simulink model "uz_d_inverter_adapter"  (R2024b)
settings: Solver=FixedStepDiscrete  StartTime=0.0  StopTime=300e-5  RelTol=1e-3
values from neighbouring files (symbols this model uses):
  t_clk = 1/f_clk    (= 1e-08)    [uz_d_inverter_adapter_init.m]
  t_clk_sig = 1/f_clk_sig    (= 0.0001)    [uz_d_inverter_adapter_init.m]
libraries: hdlsllib x12, simulink x6
settings Model: DataTypeOverride=Off  Creator=Michael Hoerner  LastModifiedBy=hufnagelde
settings SolverCC: AlgebraicLoopSolver=TrustRegion
settings DataIOCC: LimitDataPoints=on  SaveOutput=off  SaveTime=off
settings OptimizationCC: BlockReduction=off  ConditionallyExecuteInputs=off  DefaultParameterBehavior=Inlined  LifeSpan=inf
settings DebuggingCC: AlgebraicLoopMsg=error  SingleTaskRateTransMsg=warning  UnconnectedInputMsg=warning  UnconnectedOutputMsg=warning  UnconnectedLineMsg=warning  AllowSymbolicDim=off  StrictBusMsg=ErrorOnBusTreatedAsVector  SFUnexpectedBacktrackingDiag=warning  SFNoUnconditionalDefaultTransitionDiag=warning  SFExecutionAtInitializationDiag=none  ArithmeticOperatorsInVariantConditions=warning
settings HardwareCC: ProdBitPerPointer=32  ProdBitPerSizeT=32  ProdBitPerPtrDiffT=32  ProdLargestAtomicFloat=None  ProdIntDivRoundTo=Undefined  ProdEndianess=Unspecified  ProdWordSize=32  ProdHWDeviceType=ASIC/FPGA->ASIC/FPGA  ProdEqTarget=off
settings ModelReferenceCC: EnableRefExpFcnMdlSchedulingChecks=on
settings SFSimCC: SimUseLocalCustomCode=off  CustomCodeUndefinedFunction=UseInterfaceOnly
settings RTWCC: RTWUseLocalCustomCode=off  GPUComputeCapability=3.5  DLArmComputeVersion=19.05
settings CodeAppCC: StateflowObjectComments=on
settings GRTTargetCC: TargetLangStandard=C89/C90 (ANSI)
settings ConfigComp: CovScope=ReferencedModels  CovMetricSettings=dw  CovSaveCumulativeToWorkspaceVar=on  CovSaveSingleToWorkspaceVar=on  CovExternalEMLEnable=off  CovSFcnEnable=off

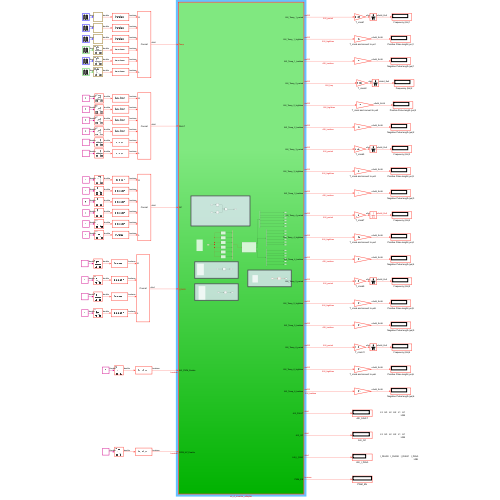
[thumbnail: Simulink's stored preview of the top-level diagram]
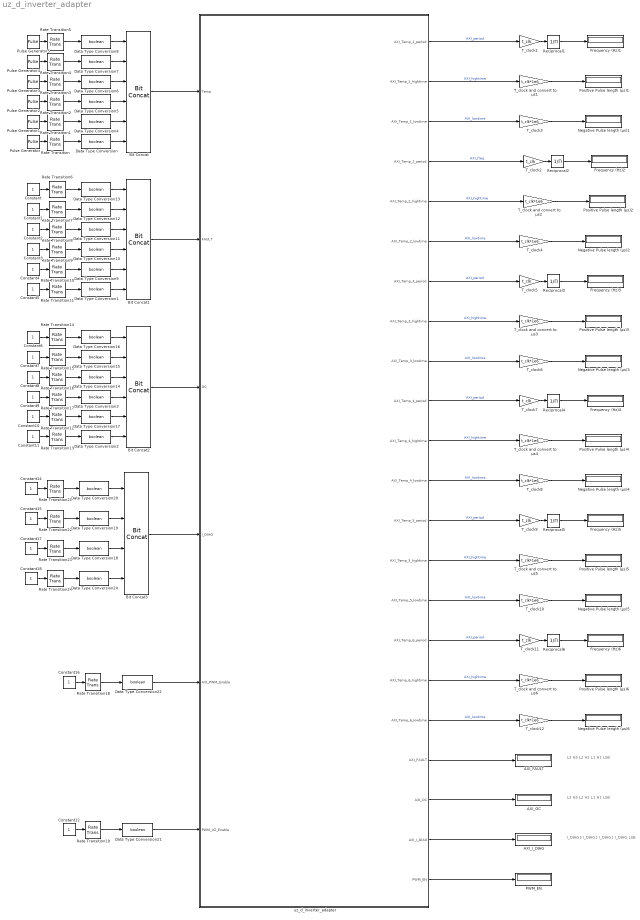
== system uz_d_inverter_adapter ==
  note: L3   H3   L2   H2   L1   H1
      |                                   LSB
  note: L3   H3   L2   H2   L1   H1
      |                                   LSB
  note: I_DIAG3   I_DIAG2   I_DIAG1   I_DIAG
      |                                                        LSB
  AXI_FAULT : Display
      settings: Format=binary (Stored Integer)
  AXI_I_DIAG : Display
      settings: Format=binary (Stored Integer)
  AXI_OC : Display
      settings: Format=binary (Stored Integer)
  Bit Concat : hdlsllib/Logic and Bit Operations/Bit Concat  numInputs=6
  Bit Concat1 : hdlsllib/Logic and Bit Operations/Bit Concat  numInputs=6
  Bit Concat2 : hdlsllib/Logic and Bit Operations/Bit Concat  numInputs=6
  Bit Concat3 : hdlsllib/Logic and Bit Operations/Bit Concat  numInputs=4
  Constant{,1..12,14..18} (18 alike) : Constant
  Data Type Conversion{,1..22,24} (24 alike) : DataTypeConversion  OutDataTypeStr=boolean  SaturateOnIntegerOverflow=off  RndMeth=Floor
  Frequency (Hz){1..6} (6 alike) : Display
  Negative Pulse length (µs){1..6} (6 alike) : Display
  PWM_EN : Display
      settings: Format=decimal (Stored Integer)
  Positive Pulse length (µs){1..6} (6 alike) : Display
  Pulse Generator : DiscretePulseGenerator  PulseType=Time based  Period=t_clk_sig  PulseWidth=10
  Pulse Generator1 : DiscretePulseGenerator  PulseType=Time based  Period=t_clk_sig  PulseWidth=20
  Pulse Generator2 : DiscretePulseGenerator  PulseType=Time based  Period=t_clk_sig  PulseWidth=30
  Pulse Generator3 : DiscretePulseGenerator  PulseType=Time based  Period=t_clk_sig  PulseWidth=40
  Pulse Generator4 : DiscretePulseGenerator  PulseType=Time based  Period=t_clk_sig  PulseWidth=50
  Pulse Generator5 : DiscretePulseGenerator  PulseType=Time based  Period=t_clk_sig  PulseWidth=60
  Rate Transition{,1..5} (6 alike) : RateTransition  Deterministic=off  OutPortSampleTime=t_clk
  Rate Transition{6..19,21..24} (18 alike) : RateTransition  OutPortSampleTime=t_clk
  Reciprocal{1..6} (6 alike) : Product  Inputs=/
  T_clock and convert to µs{1..6} (6 alike) : Gain  Gain=t_clk*1e6
  T_clock{1..2,5,7,9,11} (6 alike) : Gain  Gain=t_clk
  T_clock{3..4,6,8,10,12} (6 alike) : Gain  Gain=t_clk*1e6
  uz_d_inverter_adapter : Subsystem  TreatAsAtomicUnit=on
  wires:
  Pulse Generator/1 -> Rate Transition/1
  Pulse Generator1/1 -> Rate Transition1/1
  Pulse Generator2/1 -> Rate Transition2/1
  Pulse Generator3/1 -> Rate Transition3/1
  Pulse Generator4/1 -> Rate Transition4/1
  Pulse Generator5/1 -> Rate Transition5/1
  Rate Transition/1 -> Data Type Conversion/1
  Constant/1 -> Rate Transition6/1
  Constant1/1 -> Rate Transition7/1
  Constant2/1 -> Rate Transition8/1
  Constant3/1 -> Rate Transition9/1
  Constant4/1 -> Rate Transition10/1
  Constant5/1 -> Rate Transition11/1
  T_clock and convert to µs1/1 -> Positive Pulse length (µs)1/1
  T_clock3/1 -> Negative Pulse length (µs)1/1
  Reciprocal1/1 -> Frequency (Hz)1/1
  uz_d_inverter_adapter/3(AXI_Temp_1_lowtime) -> T_clock3/1  "AXI_lowtime"
  uz_d_inverter_adapter/2(AXI_Temp_1_hightime) -> T_clock and convert to µs1/1  "AXI_hightime"
  T_clock1/1 -> Reciprocal1/1
  uz_d_inverter_adapter/1(AXI_Temp_1_period) -> T_clock1/1  "AXI_period"
  uz_d_inverter_adapter/6(AXI_Temp_2_lowtime) -> T_clock4/1  "AXI_lowtime"
  T_clock2/1 -> Reciprocal2/1
  Reciprocal2/1 -> Frequency (Hz)2/1
  T_clock4/1 -> Negative Pulse length (µs)2/1
  uz_d_inverter_adapter/5(AXI_Temp_2_hightime) -> T_clock and convert to µs2/1  "AXI_hightime"
  T_clock and convert to µs2/1 -> Positive Pulse length (µs)2/1
  uz_d_inverter_adapter/4(AXI_Temp_2_period) -> T_clock2/1  "AXI_freq"
  uz_d_inverter_adapter/9(AXI_Temp_3_lowtime) -> T_clock6/1  "AXI_lowtime"
  T_clock5/1 -> Reciprocal3/1
  Reciprocal3/1 -> Frequency (Hz)3/1
  T_clock6/1 -> Negative Pulse length (µs)3/1
  uz_d_inverter_adapter/8(AXI_Temp_3_hightime) -> T_clock and convert to µs3/1  "AXI_hightime"
  T_clock and convert to µs3/1 -> Positive Pulse length (µs)3/1
  uz_d_inverter_adapter/7(AXI_Temp_3_period) -> T_clock5/1  "AXI_period"
  uz_d_inverter_adapter/12(AXI_Temp_4_lowtime) -> T_clock8/1  "AXI_lowtime"
  T_clock7/1 -> Reciprocal4/1
  Reciprocal4/1 -> Frequency (Hz)4/1
  T_clock8/1 -> Negative Pulse length (µs)4/1
  uz_d_inverter_adapter/11(AXI_Temp_4_hightime) -> T_clock and convert to µs4/1  "AXI_hightime"
  T_clock and convert to µs4/1 -> Positive Pulse length (µs)4/1
  uz_d_inverter_adapter/10(AXI_Temp_4_period) -> T_clock7/1  "AXI_period"
  uz_d_inverter_adapter/15(AXI_Temp_5_lowtime) -> T_clock10/1  "AXI_lowtime"
  T_clock9/1 -> Reciprocal5/1
  Reciprocal5/1 -> Frequency (Hz)5/1
  T_clock10/1 -> Negative Pulse length (µs)5/1
  uz_d_inverter_adapter/14(AXI_Temp_5_hightime) -> T_clock and convert to µs5/1  "AXI_hightime"
  T_clock and convert to µs5/1 -> Positive Pulse length (µs)5/1
  uz_d_inverter_adapter/13(AXI_Temp_5_period) -> T_clock9/1  "AXI_period"
  uz_d_inverter_adapter/18(AXI_Temp_6_lowtime) -> T_clock12/1  "AXI_lowtime"
  T_clock11/1 -> Reciprocal6/1
  Reciprocal6/1 -> Frequency (Hz)6/1
  T_clock12/1 -> Negative Pulse length (µs)6/1
  uz_d_inverter_adapter/17(AXI_Temp_6_hightime) -> T_clock and convert to µs6/1  "AXI_hightime"
  T_clock and convert to µs6/1 -> Positive Pulse length (µs)6/1
  uz_d_inverter_adapter/16(AXI_Temp_6_period) -> T_clock11/1  "AXI_period"
  uz_d_inverter_adapter/19(AXI_FAULT) -> AXI_FAULT/1
  Data Type Conversion5/1 -> Bit Concat/4
  Data Type Conversion6/1 -> Bit Concat/3
  Data Type Conversion7/1 -> Bit Concat/2
  Data Type Conversion8/1 -> Bit Concat/1
  Constant16/1 -> Rate Transition18/1
  Rate Transition18/1 -> Data Type Conversion22/1
  Bit Concat/1 -> uz_d_inverter_adapter/1(Temp)
  Rate Transition1/1 -> Data Type Conversion4/1
  Rate Transition2/1 -> Data Type Conversion5/1
  Rate Transition3/1 -> Data Type Conversion6/1
  Rate Transition4/1 -> Data Type Conversion7/1
  Rate Transition5/1 -> Data Type Conversion8/1
  Data Type Conversion/1 -> Bit Concat/6
  Data Type Conversion4/1 -> Bit Concat/5
  Data Type Conversion11/1 -> Bit Concat1/3
  Data Type Conversion10/1 -> Bit Concat1/4
  Data Type Conversion9/1 -> Bit Concat1/5
  Data Type Conversion12/1 -> Bit Concat1/2
  Data Type Conversion13/1 -> Bit Concat1/1
  Data Type Conversion1/1 -> Bit Concat1/6
  Bit Concat1/1 -> uz_d_inverter_adapter/2(FAULT)
  Rate Transition6/1 -> Data Type Conversion13/1
  Rate Transition7/1 -> Data Type Conversion12/1
  Rate Transition8/1 -> Data Type Conversion11/1
  Rate Transition9/1 -> Data Type Conversion10/1
  Rate Transition10/1 -> Data Type Conversion9/1
  Rate Transition11/1 -> Data Type Conversion1/1
  Data Type Conversion22/1 -> uz_d_inverter_adapter/5(AXI_PWM_Enable)
  Data Type Conversion16/1 -> Bit Concat2/1
  Rate Transition16/1 -> Data Type Conversion14/1
  Rate Transition17/1 -> Data Type Conversion3/1
  Rate Transition14/1 -> Data Type Conversion16/1
  Rate Transition13/1 -> Data Type Conversion2/1
  Data Type Conversion3/1 -> Bit Concat2/4
  Data Type Conversion14/1 -> Bit Concat2/3
  Data Type Conversion15/1 -> Bit Concat2/2
  Rate Transition12/1 -> Data Type Conversion17/1
  Constant6/1 -> Rate Transition14/1
  Constant8/1 -> Rate Transition16/1
  Constant11/1 -> Rate Transition13/1
  Constant10/1 -> Rate Transition12/1
  Data Type Conversion17/1 -> Bit Concat2/5
  Constant9/1 -> Rate Transition17/1
  Rate Transition15/1 -> Data Type Conversion15/1
  Constant7/1 -> Rate Transition15/1
  Data Type Conversion2/1 -> Bit Concat2/6
  Bit Concat2/1 -> uz_d_inverter_adapter/3(OC)
  Constant18/1 -> Rate Transition24/1
  Constant15/1 -> Rate Transition22/1
  Rate Transition22/1 -> Data Type Conversion19/1
  Constant14/1 -> Rate Transition21/1
  Constant17/1 -> Rate Transition23/1
  Rate Transition24/1 -> Data Type Conversion24/1
  Rate Transition21/1 -> Data Type Conversion20/1
  Rate Transition23/1 -> Data Type Conversion18/1
  Data Type Conversion20/1 -> Bit Concat3/1
  Data Type Conversion19/1 -> Bit Concat3/2
  Data Type Conversion18/1 -> Bit Concat3/3
  Data Type Conversion24/1 -> Bit Concat3/4
  Bit Concat3/1 -> uz_d_inverter_adapter/4(I_DIAG)
  uz_d_inverter_adapter/20(AXI_OC) -> AXI_OC/1
  uz_d_inverter_adapter/21(AXI_I_DIAG) -> AXI_I_DIAG/1
  uz_d_inverter_adapter/22(PWM_EN) -> PWM_EN/1
  Constant12/1 -> Rate Transition19/1
  Rate Transition19/1 -> Data Type Conversion21/1
  Data Type Conversion21/1 -> uz_d_inverter_adapter/6(PWM_UZ_Enable)

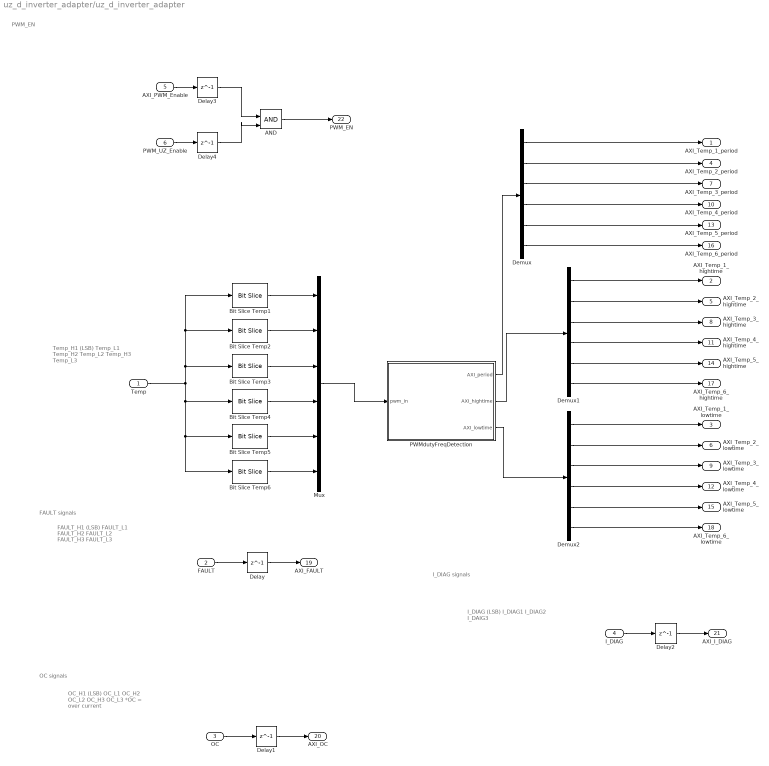
== system uz_d_inverter_adapter/uz_d_inverter_adapter ==
  note: OC signals
  note: Temp_H1   (LSB)
      |
      | Temp_L1
      |
      | Temp_H2
      |
      | Temp_L2
      |
      | Temp_H3
      |
      | Temp_L3
  note: FAULT_H1   (LSB)
      |
      | FAULT_L1
      |
      | FAULT_H2
      |
      | FAULT_L2
      |
      | FAULT_H3
      |
      | FAULT_L3
  note: OC_H1   (LSB)
      |
      | OC_L1
      |
      | OC_H2
      |
      | OC_L2
      |
      | OC_H3
      |
      | OC_L3
      |
      | *OC = over current
  note: I_DIAG   (LSB)
      |
      | I_DIAG1
      |
      | I_DIAG2
      |
      | I_DAIG3
  note: FAULT signals
  note: I_DIAG signals
  note: PWM_EN
  Temp : Inport
  FAULT : Inport  Port=2
  OC : Inport  Port=3
  I_DIAG : Inport  Port=4
  AXI_PWM_Enable : Inport  Port=5  OutDataTypeStr=boolean
  PWM_UZ_Enable : Inport  Port=6  OutDataTypeStr=boolean
  AND : Logic  IconShape=distinctive  AllPortsSameDT=off  OutDataTypeStr=boolean
  Bit Slice Temp1 : hdlsllib/Logic and Bit Operations/Bit Slice  lidx=0  ridx=0
  Bit Slice Temp2 : hdlsllib/Logic and Bit Operations/Bit Slice  lidx=1  ridx=1
  Bit Slice Temp3 : hdlsllib/Logic and Bit Operations/Bit Slice  lidx=2  ridx=2
  Bit Slice Temp4 : hdlsllib/Logic and Bit Operations/Bit Slice  lidx=3  ridx=3
  Bit Slice Temp5 : hdlsllib/Logic and Bit Operations/Bit Slice  lidx=4  ridx=4
  Bit Slice Temp6 : hdlsllib/Logic and Bit Operations/Bit Slice  lidx=5  ridx=5
  Delay{,1..4} (5 alike) : Delay  DelayLength=1
  Demux : Demux  Outputs=6
  Demux1 : Demux  Outputs=6
  Demux2 : Demux  Outputs=6
  Mux : Mux  Inputs=6
  PWMdutyFreqDetection : Subsystem  TreatAsAtomicUnit=on
  AXI_Temp_1_period : Outport  PortDimensions=1  VectorParamsAs1DForOutWhenUnconnected=off
  AXI_Temp_1_hightime : Outport  Port=2  PortDimensions=1  VectorParamsAs1DForOutWhenUnconnected=off
  AXI_Temp_1_lowtime : Outport  Port=3  PortDimensions=1  VectorParamsAs1DForOutWhenUnconnected=off
  AXI_Temp_2_period : Outport  Port=4  PortDimensions=1  VectorParamsAs1DForOutWhenUnconnected=off
  AXI_Temp_2_hightime : Outport  Port=5  PortDimensions=1  VectorParamsAs1DForOutWhenUnconnected=off
  AXI_Temp_2_lowtime : Outport  Port=6  PortDimensions=1  VectorParamsAs1DForOutWhenUnconnected=off
  AXI_Temp_3_period : Outport  Port=7  PortDimensions=1  VectorParamsAs1DForOutWhenUnconnected=off
  AXI_Temp_3_hightime : Outport  Port=8  PortDimensions=1  VectorParamsAs1DForOutWhenUnconnected=off
  AXI_Temp_3_lowtime : Outport  Port=9  PortDimensions=1  VectorParamsAs1DForOutWhenUnconnected=off
  AXI_Temp_4_period : Outport  Port=10  PortDimensions=1  VectorParamsAs1DForOutWhenUnconnected=off
  AXI_Temp_4_hightime : Outport  Port=11  PortDimensions=1  VectorParamsAs1DForOutWhenUnconnected=off
  AXI_Temp_4_lowtime : Outport  Port=12  PortDimensions=1  VectorParamsAs1DForOutWhenUnconnected=off
  AXI_Temp_5_period : Outport  Port=13  PortDimensions=1  VectorParamsAs1DForOutWhenUnconnected=off
  AXI_Temp_5_hightime : Outport  Port=14  PortDimensions=1  VectorParamsAs1DForOutWhenUnconnected=off
  AXI_Temp_5_lowtime : Outport  Port=15  PortDimensions=1  VectorParamsAs1DForOutWhenUnconnected=off
  AXI_Temp_6_period : Outport  Port=16  PortDimensions=1  VectorParamsAs1DForOutWhenUnconnected=off
  AXI_Temp_6_hightime : Outport  Port=17  PortDimensions=1  VectorParamsAs1DForOutWhenUnconnected=off
  AXI_Temp_6_lowtime : Outport  Port=18  PortDimensions=1  VectorParamsAs1DForOutWhenUnconnected=off
  AXI_FAULT : Outport  Port=19  PortDimensions=1  VectorParamsAs1DForOutWhenUnconnected=off
  AXI_OC : Outport  Port=20  PortDimensions=1  VectorParamsAs1DForOutWhenUnconnected=off
  AXI_I_DIAG : Outport  Port=21  PortDimensions=1  VectorParamsAs1DForOutWhenUnconnected=off
  PWM_EN : Outport  Port=22  PortDimensions=1  VectorParamsAs1DForOutWhenUnconnected=off
  wires:
  OC/1 -> Delay1/1
  I_DIAG/1 -> Delay2/1
  AXI_PWM_Enable/1 -> Delay3/1
  AND/1 -> PWM_EN/1
  Delay2/1 -> AXI_I_DIAG/1
  Delay1/1 -> AXI_OC/1
  PWMdutyFreqDetection/1(AXI_period) -> Demux/1
  PWMdutyFreqDetection/2(AXI_hightime) -> Demux1/1
  PWMdutyFreqDetection/3(AXI_lowtime) -> Demux2/1
  Demux/1 -> AXI_Temp_1_period/1
  Demux1/1 -> AXI_Temp_1_hightime/1
  Demux2/1 -> AXI_Temp_1_lowtime/1
  Demux/2 -> AXI_Temp_2_period/1
  Demux/3 -> AXI_Temp_3_period/1
  Demux/4 -> AXI_Temp_4_period/1
  Demux/5 -> AXI_Temp_5_period/1
  Demux/6 -> AXI_Temp_6_period/1
  Demux1/3 -> AXI_Temp_3_hightime/1
  Demux2/3 -> AXI_Temp_3_lowtime/1
  Demux1/2 -> AXI_Temp_2_hightime/1
  Demux2/2 -> AXI_Temp_2_lowtime/1
  Demux1/4 -> AXI_Temp_4_hightime/1
  Demux1/6 -> AXI_Temp_6_hightime/1
  Demux2/6 -> AXI_Temp_6_lowtime/1
  Demux2/4 -> AXI_Temp_4_lowtime/1
  Demux1/5 -> AXI_Temp_5_hightime/1
  Demux2/5 -> AXI_Temp_5_lowtime/1
  Temp/1 -> Bit Slice Temp6/1, Bit Slice Temp5/1, Bit Slice Temp4/1, Bit Slice Temp2/1, Bit Slice Temp1/1, Bit Slice Temp3/1
  Bit Slice Temp2/1 -> Mux/2
  Bit Slice Temp3/1 -> Mux/3
  Bit Slice Temp4/1 -> Mux/4
  Bit Slice Temp5/1 -> Mux/5
  Bit Slice Temp6/1 -> Mux/6
  Bit Slice Temp1/1 -> Mux/1
  Delay/1 -> AXI_FAULT/1
  FAULT/1 -> Delay/1
  Mux/1 -> PWMdutyFreqDetection/1(pwm_in)
  PWM_UZ_Enable/1 -> Delay4/1
  Delay3/1 -> AND/1
  Delay4/1 -> AND/2

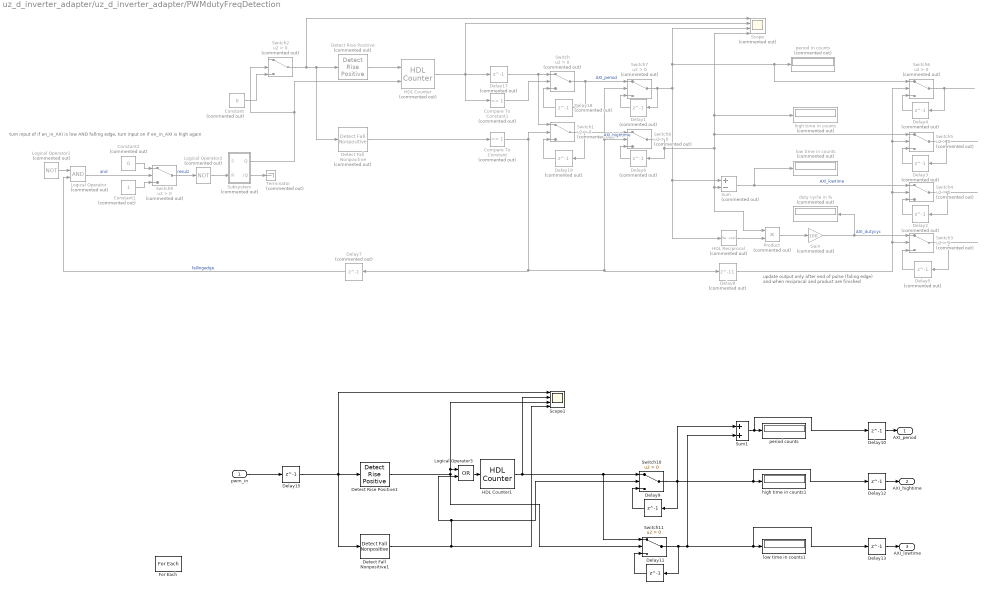
== system uz_d_inverter_adapter/uz_d_inverter_adapter/PWMdutyFreqDetection ==
  note: turn input of if en_in_AXI is low AND falling edge, turn input on if en_in_AXI is high again
  note: update output only after end of pulse (faling edge)
      | and when reciprocal and product are finished
  pwm_in : Inport  Partition=on  PartitionDimension=1  PartitionWidth=1  PartitionOffset=0
  Compare To Constant : simulink/Logic and Bit Operations/Compare To Constant  Commented=on  relop===  const=1  OutDataTypeStr=boolean
  Compare To Constant1 : simulink/Logic and Bit Operations/Compare To Constant  Commented=on  relop===  const=1  OutDataTypeStr=boolean
  Constant : Constant  Commented=on  Value=0  OutDataTypeStr=boolean  SampleTime=-1
  Constant1 : Constant  Commented=on  OutDataTypeStr=boolean  SampleTime=-1
  Constant2 : Constant  Commented=on  Value=0  OutDataTypeStr=boolean  SampleTime=-1
  Delay{1..7,17..19} (10 alike) : Delay  Commented=on  DelayLength=1
  Delay{9..13,15} (6 alike) : Delay  DelayLength=1
  Delay8 : Delay  Commented=on  DelayLength=11
  Detect Fall Nonpositive : simulink/Logic and Bit Operations/Detect Fall Nonpositive  Commented=on  vinit=0  OutDataTypeStr=boolean
  Detect Fall Nonpositive1 : simulink/Logic and Bit Operations/Detect Fall Nonpositive  vinit=0  OutDataTypeStr=boolean
  Detect Rise Positive : simulink/Logic and Bit Operations/Detect Rise Positive  Commented=on  vinit=0  OutDataTypeStr=boolean
  Detect Rise Positive1 : simulink/Logic and Bit Operations/Detect Rise Positive  vinit=0  OutDataTypeStr=boolean
  For Each : ForEach  DisableCoverage=on
  Gain : Gain  Commented=on  Gain=100  OutDataTypeStr=fixdt(1,32,24)
  HDL Counter : hdlsllib/Sources/HDL Counter  Commented=on  CountType=Count limited  CountInit=1  CountStep=1  CountMax=2500000  CountFromType=Specify  CountFrom=1  CountResetPort=on  CountLoadPort=off  CountEnbPort=on  CountDirPort=off  CountHitOutputPort=off  CountDataType=Unsigned  CountWordLen=32  CountFracLen=0  CountSampTime=1
  HDL Counter1 : hdlsllib/Sources/HDL Counter  CountType=Count limited  CountInit=1  CountStep=1  CountMax=2500000  CountFromType=Specify  CountFrom=1  CountResetPort=on  CountLoadPort=off  CountEnbPort=off  CountDirPort=off  CountHitOutputPort=off  CountDataType=Unsigned  CountWordLen=32  CountFracLen=0  CountSampTime=1
  HDL Reciprocal : Reciprocal  Commented=on
  Logical Operator : Logic  Commented=on  AllPortsSameDT=off  OutDataTypeStr=boolean
  Logical Operator1 : Logic  Commented=on  Operator=NOT  AllPortsSameDT=off  OutDataTypeStr=boolean
  Logical Operator2 : Logic  Commented=on  Operator=NOT  AllPortsSameDT=off  OutDataTypeStr=boolean
  Logical Operator3 : Logic  Operator=OR  AllPortsSameDT=off  OutDataTypeStr=boolean
  Product : Product  Commented=on  OutDataTypeStr=fixdt(1,32,30)
  Scope : Scope  Commented=on  NumInputPorts=4
  Scope1 : Scope  NumInputPorts=4
  Subsystem : Subsystem  Commented=on
  Sum : Sum  Commented=on  Inputs=+-  AccumDataTypeStr=uint32
  Sum1 : Sum  AccumDataTypeStr=uint32
  Switch{,1..9} (10 alike) : Switch  Commented=on  Criteria=u2 > Threshold  SaturateOnIntegerOverflow=off  InputSameDT=off
  Switch10 : Switch  Criteria=u2 > Threshold  SaturateOnIntegerOverflow=off  InputSameDT=off
  Switch11 : Switch  Criteria=u2 > Threshold  SaturateOnIntegerOverflow=off  InputSameDT=off
  Terminator : Terminator  Commented=on
  duty cycle in % : Display  Commented=on
  high time in counts : Display  Commented=on
  high time in counts1 : Display
  low time in counts : Display  Commented=on
  low time in counts1 : Display
  period counts : Display
  period in counts : Display  Commented=on
  AXI_period : Outport  ConcatenationDimension=1
  AXI_hightime : Outport  Port=2  ConcatenationDimension=1
  AXI_lowtime : Outport  Port=3  ConcatenationDimension=1
  wires:
  Detect Rise Positive/1 -> HDL Counter/1
  Switch1/1 -> Delay19/1, Switch8/1  "AXI_hightime"
  Delay17/1 -> Switch1/1, Switch/1
  Switch2/1 -> Scope/1, Detect Fall Nonpositive/1, Detect Rise Positive/1
  Detect Fall Nonpositive/1 -> Compare To Constant/1
  HDL Counter/1 -> Scope/2, Compare To Constant1/1, Delay17/1
  Product/1 -> Gain/1
  Gain/1 -> Switch3/1, duty cycle in %/1  "AXI_dutycyc"
  Sum/1 -> Switch4/1, low time in counts/1  "AXI_lowtime"
  Delay18/1 -> Switch/3
  Switch/1 -> Delay18/1, Switch7/1  "AXI_period"
  Compare To Constant1/1 -> Switch/2
  Delay19/1 -> Switch1/3
  Compare To Constant/1 -> Delay7/1, Switch7/2, Switch8/2, Delay8/1, Switch1/2
  Switch3/1 -> Delay5/1
  Switch4/1 -> Delay2/1
  Switch5/1 -> Delay3/1
  Switch6/1 -> Delay4/1
  HDL Reciprocal/1 -> Product/2
  ? -> Switch2/1
  Delay5/1 -> Switch3/3
  Delay4/1 -> Switch6/3
  Delay3/1 -> Switch5/3
  Delay2/1 -> Switch4/3
  Constant/1 -> Switch2/3
  ? -> Logical Operator1/1, Subsystem/1(S)  "en"
  Switch7/1 -> Delay1/1, HDL Reciprocal/1, Sum/1, Scope/3, Switch6/1, period in counts/1
  Delay1/1 -> Switch7/3
  Switch8/1 -> Delay6/1, Switch5/1, high time in counts/1, Scope/4, Product/1, Sum/2
  Delay6/1 -> Switch8/3
  Delay7/1 -> Logical Operator/2  "fallingedge"
  Constant1/1 -> Switch9/3
  Constant2/1 -> Switch9/1
  Logical Operator1/1 -> Logical Operator/1
  Logical Operator/1 -> Switch9/2  "and"
  Switch9/1 -> Logical Operator2/1  "resulz"
  Logical Operator2/1 -> Subsystem/2(R)
  Subsystem/1(Q) -> HDL Counter/2, Switch2/2
  Subsystem/2(!Q) -> Terminator/1
  Delay8/1 -> Switch6/2, Switch5/2, Switch4/2, Switch3/2
  Logical Operator3/1 -> HDL Counter1/1
  Sum1/1 -> Delay10/1, period counts/1
  Detect Fall Nonpositive1/1 -> Logical Operator3/2, Switch10/2, Scope1/4
  Delay12/1 -> AXI_hightime/1
  Delay10/1 -> AXI_period/1
  Delay9/1 -> Switch10/3
  Delay11/1 -> Switch11/3
  HDL Counter1/1 -> Switch11/1, Switch10/1, Scope1/2
  Detect Rise Positive1/1 -> Switch11/2, Logical Operator3/1, Scope1/3
  Delay13/1 -> AXI_lowtime/1
  Delay15/1 -> Detect Fall Nonpositive1/1, Scope1/1, Detect Rise Positive1/1
  pwm_in/1 -> Delay15/1
  Switch10/1 -> Sum1/1, Delay12/1, high time in counts1/1, Delay9/1
  Switch11/1 -> Sum1/2, Delay13/1, low time in counts1/1, Delay11/1

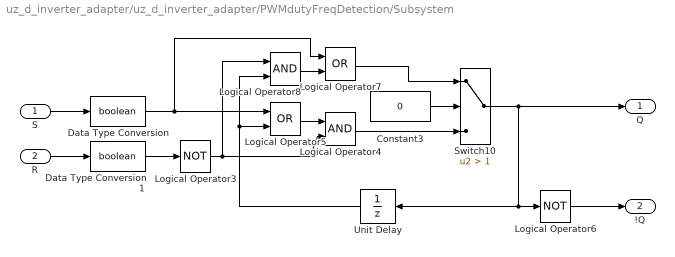
== system uz_d_inverter_adapter/uz_d_inverter_adapter/PWMdutyFreqDetection/Subsystem ==
  S : Inport
  R : Inport  Port=2
  Constant3 : Constant  Value=0  OutDataTypeStr=boolean  SampleTime=-1
  Data Type Conversion : DataTypeConversion  OutDataTypeStr=boolean  SaturateOnIntegerOverflow=off  RndMeth=Floor
  Data Type Conversion1 : DataTypeConversion  OutDataTypeStr=boolean  SaturateOnIntegerOverflow=off  RndMeth=Floor
  Logical Operator3 : Logic  Operator=NOT  AllPortsSameDT=off  OutDataTypeStr=boolean
  Logical Operator4 : Logic  AllPortsSameDT=off  OutDataTypeStr=boolean
  Logical Operator5 : Logic  Operator=OR  AllPortsSameDT=off  OutDataTypeStr=boolean
  Logical Operator6 : Logic  Operator=NOT  AllPortsSameDT=off  OutDataTypeStr=boolean
  Logical Operator7 : Logic  Operator=OR  AllPortsSameDT=off  OutDataTypeStr=boolean
  Logical Operator8 : Logic  AllPortsSameDT=off  OutDataTypeStr=boolean
  Switch10 : Switch  Criteria=u2 > Threshold  Threshold=1  SaturateOnIntegerOverflow=off  InputSameDT=off
  Unit Delay : UnitDelay  SampleTime=-1  HasFrameUpgradeWarning=on
  Q : Outport
  !Q : Outport  Port=2
  wires:
  Logical Operator4/1 -> Switch10/3
  Data Type Conversion/1 -> Logical Operator5/1, Logical Operator7/1
  Unit Delay/1 -> Logical Operator5/2, Logical Operator8/2
  Logical Operator3/1 -> Logical Operator4/2, Logical Operator8/1
  R/1 -> Data Type Conversion1/1
  S/1 -> Data Type Conversion/1
  Constant3/1 -> Switch10/2
  Logical Operator7/1 -> Switch10/1
  Logical Operator8/1 -> Logical Operator7/2
  Data Type Conversion1/1 -> Logical Operator3/1
  Switch10/1 -> Q/1, Unit Delay/1, Logical Operator6/1
  Logical Operator5/1 -> Logical Operator4/1
  Logical Operator6/1 -> !Q/1
